simulink model "rpend_MPC2"  (R2017b)
settings: Solver=ode45  StartTime=0.0  StopTime=30  RelTol=1e-3  EnableMultiTasking=on
undefined symbols (not defined in the file): adingain, adinoffs, daoutgain, daoutoffs, h, Tres1, Tres2
libraries: simulink x4, mpclib x1
settings Model: Creator=rbabuska  LastModifiedBy=pimwu
settings DataIOCC: LimitDataPoints=on  SaveFormat=Array  SignalLoggingName=sigsOut
settings OptimizationCC: BooleanDataType=off  ExpressionDepthLimit=2147483647  InitFltsAndDblsToZero=on  LifeSpan=inf
settings DebuggingCC: SaveWithParameterizedLinksMsg=none  SignalResolutionControl=TryResolveAllWithWarning  MultiTaskDSMMsg=warning  MultiTaskCondExecSysMsg=none  AllowSymbolicDim=off  StateNameClashWarn=warning  SFUnexpectedBacktrackingDiag=warning  SFNoUnconditionalDefaultTransitionDiag=warning  SFExecutionAtInitializationDiag=none
settings HardwareCC: ProdBitPerPointer=32  ProdBitPerSizeT=32  ProdBitPerPtrDiffT=32  ProdLargestAtomicFloat=None  ProdIntDivRoundTo=Undefined  ProdEndianess=Unspecified  ProdWordSize=32  ProdHWDeviceType=32-bit Generic  TargetUnknown=on
settings ModelReferenceCC: PropagateSignalLabelsOutOfModel=off
settings CodeAppCC: StateflowObjectComments=on
settings GRTTargetCC: TargetFcnLib=ansi_tfl_tmw.mat  TargetLangStandard=C89/C90 (ANSI)  GeneratePreprocessorConditionals=Disable all  CombineOutputUpdateFcns=off  GRTInterface=on
settings ConfigComp: CovMetricSettings=dw  CovHtmlReporting=on  CovSaveCumulativeToWorkspaceVar=on  CovSaveSingleToWorkspaceVar=on  CovExternalEMLEnable=off

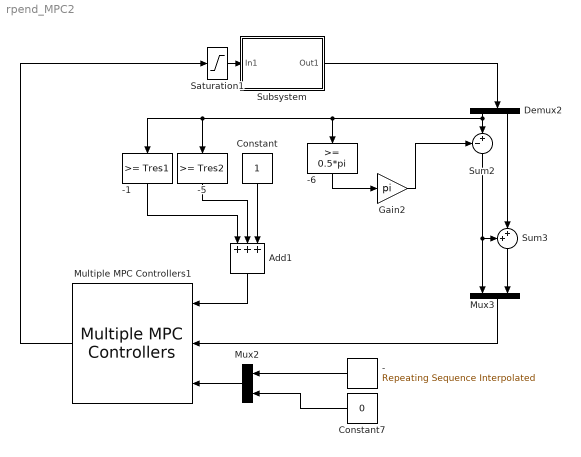
== system rpend_MPC2 ==
  - : simulink/Sources/Repeating Sequence Interpolated  OutValues=[0 0 1.5 -1.3 0 0].'  TimeValues=[0 5 10 10.2 15.5 100].'  LookUpMeth=Interpolation-Use End Values  tsamp=0.01  OutMin=[]  OutMax=[]  OutDataTypeStr=double  OutputDataTypeScalingMode=double  OutDataType=fixdt(0,8)  OutScaling=2^-10
  -1 : simulink/Logic and Bit Operations/Compare To Constant  relop=>=  const=Tres1  OutDataTypeStr=boolean
  -5 : simulink/Logic and Bit Operations/Compare To Constant  relop=>=  const=Tres2  OutDataTypeStr=boolean
  -6 : simulink/Logic and Bit Operations/Compare To Constant  relop=>=  const=0.5*pi  OutDataTypeStr=boolean
  Add1 : Sum  Inputs=+++
  Constant : Constant
  Constant7 : Constant  Value=0
  Demux2 : Demux  Outputs=2
  Gain2 : Gain  Gain=pi
  Multiple MPC Controllers1 : mpclib/Multiple MPC Controllers  mpcobjs={' mpc1',' mpc007' ,' MPC_pi0' }  x0s={'[]',' []',' []' }  Nmpc=1  theMPC=1  nmv=1  nmo=1  nmd=1  nts=1  is_designfromscratch=0  linswitch=0  ref_from_ws_multiple=off  ref_signal_name_multiple=[]  ref_preview_multiple=off  md_from_ws_multiple=off  md_signal_name_multiple=[]  md_preview_multiple=off  md_inport_multiple=off  mv_inport_multiple=off  cost_outport_multiple=off  return_sequence_multiple=off  return_qpstatus_multiple=off  return_state_multiple=off  state_inport_multiple=off  lims_inport_multiple=off  ywt_inport_multiple=off  uwt_inport_multiple=off  duwt_inport_multiple=off  rhoeps_inport_multiple=off  uref_inport_multiple=off  BlockDataType_multiple=double  SampleTimeInherited_multiple=off
      settings: SourceProductName=Model Predictive Control Toolbox  SourceProductBaseCode=MP
  Mux2 : Mux  Inputs=2
  Mux3 : Mux  Inputs=2
  Saturation1 : Saturate  UpperLimit=1  LowerLimit=-1
  Subsystem : Subsystem
      mask Display: disp('Rotational\nPendulum')
  Sum2 : Sum  Inputs=-+|
  Sum3 : Sum  Inputs=++|
  wires:
  Saturation1/1 -> Subsystem/1(In1)
  Sum2/1 -> Mux3/1, Sum3/1
  Sum3/1 -> Mux3/2
  Demux2/2 -> Sum3/2
  Add1/1 -> Multiple MPC Controllers1/1
  Mux3/1 -> Multiple MPC Controllers1/2
  Mux2/1 -> Multiple MPC Controllers1/3
  Subsystem/1(Out1) -> Demux2/1
  Constant7/1 -> Mux2/2
  Demux2/1 -> -6/1, -1/1, -5/1, Sum2/2
  -1/1 -> Add1/1
  -6/1 -> Gain2/1
  Gain2/1 -> Sum2/1
  -5/1 -> Add1/2
  Constant/1 -> Add1/3
  Multiple MPC Controllers1/1 -> Saturation1/1
  -/1 -> Mux2/1

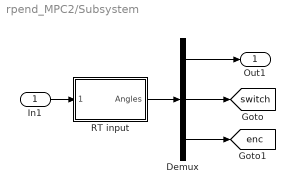
== system rpend_MPC2/Subsystem ==
  In1 : Inport
  Demux : Demux  Outputs=[2 4 1]
  RT input : Subsystem  mask{Ts=h, channels=[6 7]}
      mask prompts: Ts "Sample time [s]:"; channels "Channels to read (e.g., [6 7])"
      mask init:
      | hwinit;
      | 
      | % initialize FPGA
      | fugihandle = fugiboard('Open', 'Pendulum1');
      | fugihandle.WatchdogTimeout = 0.5;
      | fugiboard('SetParams', fugihandle);
      | fugiboard('Write', fugihandle, 0, 0, 0, 0);  % dummy write to sync interface board
      | fugiboard('Write', fugihandle, 5, 1, 0, 0);  % reset position, activate relay
      | data = fugiboard('Read', fugihandle);        % get version info from FPGA
      | % model = bitshift(data(1), -5); 
      | % version = bitand(data(1), 31);
      | % disp(sprintf('FPGA setup %d, version %d', model, version)); % for the B&P it should say 1 1, or else there is a problem
      | fugiboard('Write', fugihandle, 0, 1, 0, 0);  % end reset
      | pause(0.1);                         % give relay some time to respond
      mask Display: disp('Rotational\nPendulum')
  Out1 : Outport
  tag scope: enc=global, switch=global
  wires:
  RT input/1(Angles) -> Demux/1
  Demux/1 -> Out1/1
  Demux/2 -> [switch]
  Demux/3 -> [enc]
  In1/1 -> RT input/1(Motors)

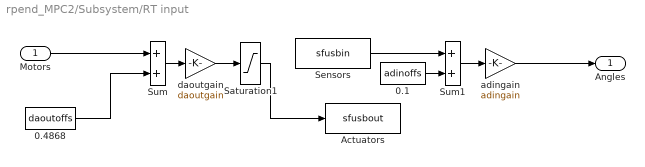
== system rpend_MPC2/Subsystem/RT input ==
  Motors : Inport
  0.1 : Constant  Value=adinoffs
  0.4868 : Constant  Value=daoutoffs
  Actuators : S-Function  FunctionName=sfusbout  Parameters=Ts, fugihandle  SFunctionDeploymentMode=off  EnableBusSupport=off
  Saturation1 : Saturate  UpperLimit=10  LowerLimit=-10
  Sensors : S-Function  FunctionName=sfusbin  Parameters=Ts, fugihandle, channels  SFunctionDeploymentMode=off  EnableBusSupport=off
  Sum : Sum  SaturateOnIntegerOverflow=on  InputSameDT=on  OutDataTypeStr=Inherit: Same as first input
  Sum1 : Sum  SaturateOnIntegerOverflow=on  InputSameDT=on  OutDataTypeStr=Inherit: Same as first input
  adingain : Gain  Gain=adingain  SaturateOnIntegerOverflow=on  OutDataTypeStr=Inherit: Same as input  ParamDataTypeStr=Inherit: Same as input
  daoutgain : Gain  Gain=daoutgain  SaturateOnIntegerOverflow=on  OutDataTypeStr=Inherit: Same as input  ParamDataTypeStr=Inherit: Same as input
  Angles : Outport
  wires:
  Sum/1 -> daoutgain/1
  0.4868/1 -> Sum/2
  Motors/1 -> Sum/1
  Sum1/1 -> adingain/1
  0.1/1 -> Sum1/2
  Sensors/1 -> Sum1/1
  adingain/1 -> Angles/1
  Saturation1/1 -> Actuators/1
  daoutgain/1 -> Saturation1/1
